simulink model "Exercise_4"  (R2024b)
settings: Solver=VariableStepAuto  StartTime=0.0  StopTime=10.0  RelTol=1e-3
settings Model: Creator=HP  LastModifiedBy=HP

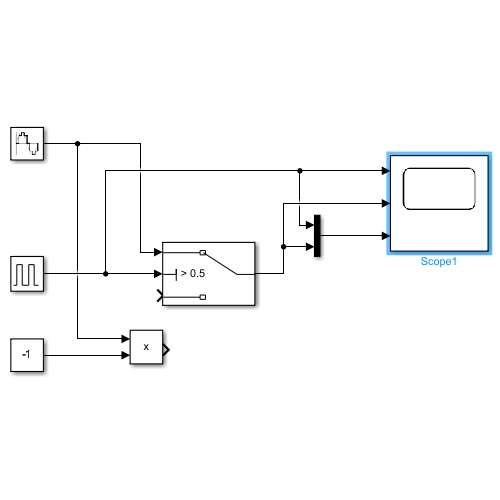
[thumbnail: Simulink's stored preview of the top-level diagram]
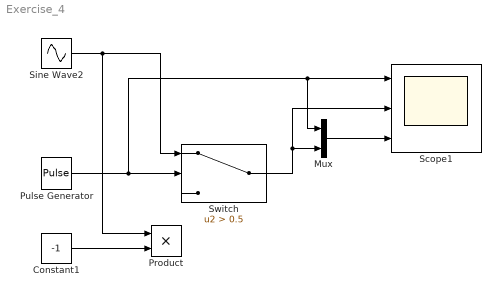
== system Exercise_4 ==
  Constant1 : Constant  Value=-1
  Mux : Mux  Inputs=2
  Product : Product
  Pulse Generator : DiscretePulseGenerator  PulseType=Time based  PulseWidth=50
  Scope1 : Scope  NumInputPorts=3
  Sine Wave2 : Sin  Frequency=20  SampleTime=0.0001
  Switch : Switch  Criteria=u2 > Threshold  Threshold=0.5  SaturateOnIntegerOverflow=off  InputSameDT=off
  wires:
  Sine Wave2/1 -> Product/1, Switch/1
  Pulse Generator/1 -> Switch/2, Mux/1, Scope1/1
  Constant1/1 -> Product/2
  Switch/1 -> Scope1/2, Mux/2
  Mux/1 -> Scope1/3
